simulink model "plant_control"  (R2023a)
settings: Solver=FixedStepAuto  StartTime=0.0  StopTime=10  FixedStep=0.01  RelTol=1e-3
values from neighbouring files (symbols this model uses):
  g = 9.81    [control_params.m]
  Ginv = inv(G)    [control_params.m]
  kF = -9.17e-5    (= -9.17e-05)    [control_params.m]
  kM = 3.24e-6    (= 3.24e-06)    [control_params.m]
  Kp_p = 7.1614    [control_params.m]
  Kp_pitch = 10.84    [control_params.m]
  Kp_q = 7.1614    [control_params.m]
  Kp_r = 3.3884    [control_params.m]
  Kp_roll = 10.84    [control_params.m]
  Kp_vx = -0.3281    [control_params.m]
  Kp_vy = 0.3281    [control_params.m]
  Kp_vz = 100    [control_params.m]
  Kp_x = 1    [control_params.m]
  Kp_y = 1    [control_params.m]
  Kp_yaw = 10.84    [control_params.m]
  Kp_z = 1    [control_params.m]
  lx = 0.4389087297    [control_params.m]
  ly = 0.4389087297    [control_params.m]
  m = 10    [control_params.m]
  Td = 1/3    (= 0.333333333333)    [control_params.m]
  Ti = 5/3    (= 1.66666666667)    [control_params.m]
libraries: slpidlib x3, shared6dof x1, simulink_extras x1, aerolibnav x1, SignalEditorBlockLib x1
settings Model: Creator=timme  LastModifiedBy=timme
settings OptimizationCC: BlockReduction=off  DefaultParameterBehavior=Inlined  BufferReuse=off

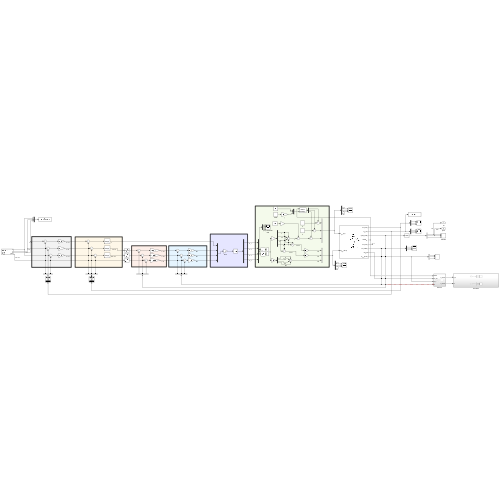
[thumbnail: Simulink's stored preview of the top-level diagram]
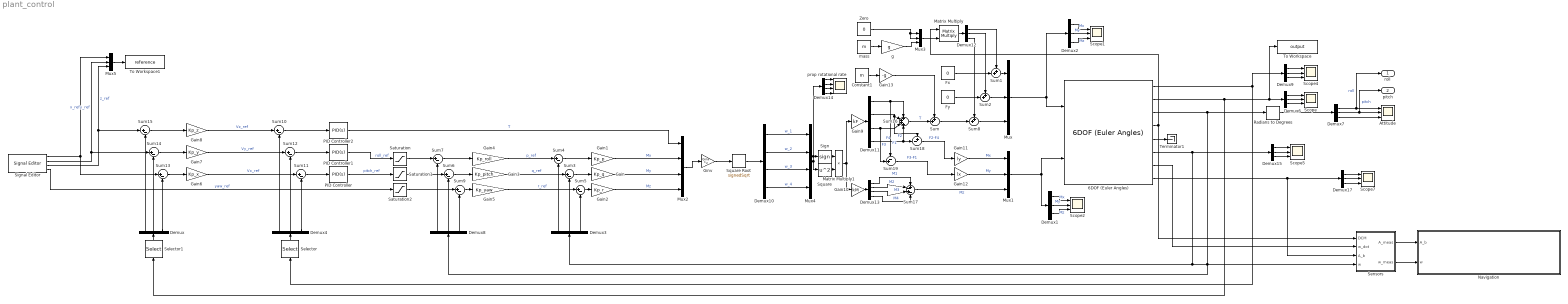
== system plant_control ==
  6DOF (Euler Angles) : shared6dof/6DOF (Euler Angles)  units=Metric (MKS)  mtype=Fixed  rep=Euler Angles  xme_0=[0 0 -1]  Vm_0=[0 0 0]  eul_0=[0 0 0]  pm_0=[0 0 0]  mass_0=m  mass_e=0.5  mass_f=2.0  inertia=I  inertia_e=eye(3)  inertia_f=2*eye(3)  k_quat=1.0  vre_flag=on  abi_flag=off  aMode=0  xme_statename=''  Vm_statename=''  eul_statename=''  quat_statename=''  pm_statename=''  mass_statename=''
  Attitude : Scope  NumInputPorts=3
  Constant1 : Constant  Value=m
  Demux{,1..4,6..9,12,15,17} (12 alike) : Demux  Outputs=3
  Demux{10..11,13..14} (4 alike) : Demux
  Fx : Constant  Value=0
  Fy : Constant  Value=0
  Gain : Gain  Gain=Kp_q
  Gain1 : Gain  Gain=Kp_p
  Gain10 : Gain  Gain=kM
  Gain11 : Gain  Gain=ly
  Gain12 : Gain  Gain=lx
  Gain13 : Gain  Gain=-g
  Gain2 : Gain  Gain=Kp_r
  Gain3 : Gain  Gain=Kp_pitch
  Gain4 : Gain  Gain=Kp_roll
  Gain5 : Gain  Gain=Kp_yaw
  Gain6 : Gain  Gain=Kp_x
  Gain7 : Gain  Gain=Kp_y
  Gain8 : Gain  Gain=Kp_z
  Gain9 : Gain  Gain=kF
  Ginv : Gain  Gain=Ginv  Multiplication=Matrix(K*u)
  Matrix Multiply : Product  Inputs=**  Multiplication=Matrix(*)
  Matrix Multiply1 : Product
  Mux{,1,3,5} (4 alike) : Mux  Inputs=3
  Mux2 : Mux
  Mux4 : Mux
  Navigation : Subsystem
  PID Controller : slpidlib/PID Controller  Controller=PID  Form=Parallel  TimeDomain=Continuous-time  UseExternalTs=off  SampleTime=-1  IntegratorMethod=Forward Euler  FilterMethod=Forward Euler  ControllerParametersSource=internal  P=Kp_vx*(1+Td/Ti)  I=Kp_vx/Ti  UseKiTs=off  D=Kp_vx*Td  N=100  UseFilter=on  TunerSelectOption=Transfer Function Based (PID Tuner App)  InitialConditionSource=internal  InitialConditionForIntegrator=0  InitialConditionForFilter=0  DifferentiatorICPrevScaledInput=0  ExternalReset=none  TrackingMode=off  Kt=1  LimitOutput=off  SatLimitsSource=internal  UpperSaturationLimit=inf  LowerSaturationLimit=-inf  LinearizeAsGain=on  AntiWindupMode=none  Kb=1  LimitIntegrator=off  UpperIntegratorSaturationLimit=inf  LowerIntegratorSaturationLimit=-inf  POutMin=[]  POutMax=[]  IOutMin=[]  IOutMax=[]  DOutMin=[]  DOutMax=[]  NOutMin=[]  NOutMax=[]  SumOutMin=[]  SumOutMax=[]  SaturationOutMin=[]  SaturationOutMax=[]  PParamMin=[]  PParamMax=[]  IParamMin=[]  IParamMax=[]  DParamMin=[]  DParamMax=[]  NParamMin=[]  NParamMax=[]  KbParamMin=[]  KbParamMax=[]  KtParamMin=[]  KtParamMax=[]  KbOutMin=[]  KbOutMax=[]  KtOutMin=[]  KtOutMax=[]  IntegratorOutMin=[]  IntegratorOutMax=[]  FilterOutMin=[]  FilterOutMax=[]  SumI1OutMin=[]  SumI1OutMax=[]  SumI2OutMin=[]  SumI2OutMax=[]  SumI3OutMin=[]  SumI3OutMax=[]  SumI4OutMin=[]  SumI4OutMax=[]  SumDOutMin=[]  SumDOutMax=[]  DifferentiatorOutMin=[]  DifferentiatorOutMax=[]  FilterDiffOutCoefMin=[]  FilterDiffOutCoefMax=[]  ReciprocalOutMin=[]  ReciprocalOutMax=[]  SumDenOutMin=[]  SumDenOutMax=[]  SumNumOutMin=[]  SumNumOutMax=[]  DivideOutMin=[]  DivideOutMax=[]  UdiffTsProdOutMin=[]  UdiffTsProdOutMax=[]  NTsProdOutMin=[]  NTsProdOutMax=[]  UintegralTsProdOutMin=[]  UintegralTsProdOutMax=[]  UngainTsProdOutMin=[]  UngainTsProdOutMax=[]  ClampingZeroOutDataTypeStr=Inherit: Inherit via back propagation  ClampingZeroOutMin=[]  ClampingZeroOutMax=[]  FilterDenConstantOutDataTypeStr=Inherit: Inherit via back propagation  FilterDenConstantOutMin=[]  FilterDenConstantOutMax=[]  PCopyOutDataTypeStr=Inherit: Inherit via back propagation  PCopyOutMin=[]  PCopyOutMax=[]  NCopyOutDataTypeStr=Inherit: Inherit via back propagation  NCopyOutMin=[]  NCopyOutMax=[]  IntegratorContinuousStateAttributes=''  IntegratorStateMustResolveToSignalObject=off  IntegratorRTWStateStorageClass=Auto  FilterContinuousStateAttributes=''  FilterStateMustResolveToSignalObject=off  FilterRTWStateStorageClass=Auto  ParallelPVariant=InternalParameters  IdealPVariant=Disabled  IVariant=InternalParameters  DVariant=InternalParameters  IntegratorVariant=Continuous  SatVariant=Disabled  AWVariant=Passthrough  PCopyVariant=Disabled  TRVariant=Disabled  FdbkBlocksVariant=Forward  IdealPFdbkVariant=Disabled  SatFdbkVariant=Disabled  DerivativeFilterVariant=ContFilter  NVariant=InternalParameters  NCopyVariant=Disabled  FilterICVariant=InternalICsFilter  IntegratorICVariant=InternalICs  ExternalResetVariant=Disabled  TRSumVariant=Passthrough  SumFdbkVariant=Disabled  SumVariant=Sum_PID  TsampFilterVariant=InternalTs  TsampNgainVariant=Passthrough  TsampIntegralVariant=Disabled_SignalSpec  ExternalSaturationOutDataTypeStr=Inherit: Same as second input
  PID Controller1 : slpidlib/PID Controller  Controller=PID  Form=Parallel  TimeDomain=Continuous-time  UseExternalTs=off  SampleTime=-1  IntegratorMethod=Forward Euler  FilterMethod=Forward Euler  ControllerParametersSource=internal  P=Kp_vy*(1+Td/Ti)  I=Kp_vy/Ti  UseKiTs=off  D=Kp_vy*Td  N=100  UseFilter=on  TunerSelectOption=Transfer Function Based (PID Tuner App)  InitialConditionSource=internal  InitialConditionForIntegrator=0  InitialConditionForFilter=0  DifferentiatorICPrevScaledInput=0  ExternalReset=none  TrackingMode=off  Kt=1  LimitOutput=off  SatLimitsSource=internal  UpperSaturationLimit=inf  LowerSaturationLimit=-inf  LinearizeAsGain=on  AntiWindupMode=none  Kb=1  LimitIntegrator=off  UpperIntegratorSaturationLimit=inf  LowerIntegratorSaturationLimit=-inf  POutMin=[]  POutMax=[]  IOutMin=[]  IOutMax=[]  DOutMin=[]  DOutMax=[]  NOutMin=[]  NOutMax=[]  SumOutMin=[]  SumOutMax=[]  SaturationOutMin=[]  SaturationOutMax=[]  PParamMin=[]  PParamMax=[]  IParamMin=[]  IParamMax=[]  DParamMin=[]  DParamMax=[]  NParamMin=[]  NParamMax=[]  KbParamMin=[]  KbParamMax=[]  KtParamMin=[]  KtParamMax=[]  KbOutMin=[]  KbOutMax=[]  KtOutMin=[]  KtOutMax=[]  IntegratorOutMin=[]  IntegratorOutMax=[]  FilterOutMin=[]  FilterOutMax=[]  SumI1OutMin=[]  SumI1OutMax=[]  SumI2OutMin=[]  SumI2OutMax=[]  SumI3OutMin=[]  SumI3OutMax=[]  SumI4OutMin=[]  SumI4OutMax=[]  SumDOutMin=[]  SumDOutMax=[]  DifferentiatorOutMin=[]  DifferentiatorOutMax=[]  FilterDiffOutCoefMin=[]  FilterDiffOutCoefMax=[]  ReciprocalOutMin=[]  ReciprocalOutMax=[]  SumDenOutMin=[]  SumDenOutMax=[]  SumNumOutMin=[]  SumNumOutMax=[]  DivideOutMin=[]  DivideOutMax=[]  UdiffTsProdOutMin=[]  UdiffTsProdOutMax=[]  NTsProdOutMin=[]  NTsProdOutMax=[]  UintegralTsProdOutMin=[]  UintegralTsProdOutMax=[]  UngainTsProdOutMin=[]  UngainTsProdOutMax=[]  ClampingZeroOutDataTypeStr=Inherit: Inherit via back propagation  ClampingZeroOutMin=[]  ClampingZeroOutMax=[]  FilterDenConstantOutDataTypeStr=Inherit: Inherit via back propagation  FilterDenConstantOutMin=[]  FilterDenConstantOutMax=[]  PCopyOutDataTypeStr=Inherit: Inherit via back propagation  PCopyOutMin=[]  PCopyOutMax=[]  NCopyOutDataTypeStr=Inherit: Inherit via back propagation  NCopyOutMin=[]  NCopyOutMax=[]  IntegratorContinuousStateAttributes=''  IntegratorStateMustResolveToSignalObject=off  IntegratorRTWStateStorageClass=Auto  FilterContinuousStateAttributes=''  FilterStateMustResolveToSignalObject=off  FilterRTWStateStorageClass=Auto  ParallelPVariant=InternalParameters  IdealPVariant=Disabled  IVariant=InternalParameters  DVariant=InternalParameters  IntegratorVariant=Continuous  SatVariant=Disabled  AWVariant=Passthrough  PCopyVariant=Disabled  TRVariant=Disabled  FdbkBlocksVariant=Forward  IdealPFdbkVariant=Disabled  SatFdbkVariant=Disabled  DerivativeFilterVariant=ContFilter  NVariant=InternalParameters  NCopyVariant=Disabled  FilterICVariant=InternalICsFilter  IntegratorICVariant=InternalICs  ExternalResetVariant=Disabled  TRSumVariant=Passthrough  SumFdbkVariant=Disabled  SumVariant=Sum_PID  TsampFilterVariant=InternalTs  TsampNgainVariant=Passthrough  TsampIntegralVariant=Disabled_SignalSpec  ExternalSaturationOutDataTypeStr=Inherit: Same as second input
  PID Controller2 : slpidlib/PID Controller  Controller=PID  Form=Parallel  TimeDomain=Continuous-time  UseExternalTs=off  SampleTime=-1  IntegratorMethod=Forward Euler  FilterMethod=Forward Euler  ControllerParametersSource=internal  P=Kp_vz  I=50  UseKiTs=off  D=0  N=100  UseFilter=on  TunerSelectOption=Transfer Function Based (PID Tuner App)  InitialConditionSource=internal  InitialConditionForIntegrator=0  InitialConditionForFilter=0  DifferentiatorICPrevScaledInput=0  ExternalReset=none  TrackingMode=off  Kt=1  LimitOutput=off  SatLimitsSource=internal  UpperSaturationLimit=inf  LowerSaturationLimit=-inf  LinearizeAsGain=on  AntiWindupMode=none  Kb=1  LimitIntegrator=off  UpperIntegratorSaturationLimit=inf  LowerIntegratorSaturationLimit=-inf  POutMin=[]  POutMax=[]  IOutMin=[]  IOutMax=[]  DOutMin=[]  DOutMax=[]  NOutMin=[]  NOutMax=[]  SumOutMin=[]  SumOutMax=[]  SaturationOutMin=[]  SaturationOutMax=[]  PParamMin=[]  PParamMax=[]  IParamMin=[]  IParamMax=[]  DParamMin=[]  DParamMax=[]  NParamMin=[]  NParamMax=[]  KbParamMin=[]  KbParamMax=[]  KtParamMin=[]  KtParamMax=[]  KbOutMin=[]  KbOutMax=[]  KtOutMin=[]  KtOutMax=[]  IntegratorOutMin=[]  IntegratorOutMax=[]  FilterOutMin=[]  FilterOutMax=[]  SumI1OutMin=[]  SumI1OutMax=[]  SumI2OutMin=[]  SumI2OutMax=[]  SumI3OutMin=[]  SumI3OutMax=[]  SumI4OutMin=[]  SumI4OutMax=[]  SumDOutMin=[]  SumDOutMax=[]  DifferentiatorOutMin=[]  DifferentiatorOutMax=[]  FilterDiffOutCoefMin=[]  FilterDiffOutCoefMax=[]  ReciprocalOutMin=[]  ReciprocalOutMax=[]  SumDenOutMin=[]  SumDenOutMax=[]  SumNumOutMin=[]  SumNumOutMax=[]  DivideOutMin=[]  DivideOutMax=[]  UdiffTsProdOutMin=[]  UdiffTsProdOutMax=[]  NTsProdOutMin=[]  NTsProdOutMax=[]  UintegralTsProdOutMin=[]  UintegralTsProdOutMax=[]  UngainTsProdOutMin=[]  UngainTsProdOutMax=[]  ClampingZeroOutDataTypeStr=Inherit: Inherit via back propagation  ClampingZeroOutMin=[]  ClampingZeroOutMax=[]  FilterDenConstantOutDataTypeStr=Inherit: Inherit via back propagation  FilterDenConstantOutMin=[]  FilterDenConstantOutMax=[]  PCopyOutDataTypeStr=Inherit: Inherit via back propagation  PCopyOutMin=[]  PCopyOutMax=[]  NCopyOutDataTypeStr=Inherit: Inherit via back propagation  NCopyOutMin=[]  NCopyOutMax=[]  IntegratorContinuousStateAttributes=''  IntegratorStateMustResolveToSignalObject=off  IntegratorRTWStateStorageClass=Auto  FilterContinuousStateAttributes=''  FilterStateMustResolveToSignalObject=off  FilterRTWStateStorageClass=Auto  ParallelPVariant=InternalParameters  IdealPVariant=Disabled  IVariant=InternalParameters  DVariant=InternalParameters  IntegratorVariant=Continuous  SatVariant=Disabled  AWVariant=Passthrough  PCopyVariant=Disabled  TRVariant=Disabled  FdbkBlocksVariant=Forward  IdealPFdbkVariant=Disabled  SatFdbkVariant=Disabled  DerivativeFilterVariant=ContFilter  NVariant=InternalParameters  NCopyVariant=Disabled  FilterICVariant=InternalICsFilter  IntegratorICVariant=InternalICs  ExternalResetVariant=Disabled  TRSumVariant=Passthrough  SumFdbkVariant=Disabled  SumVariant=Sum_PID  TsampFilterVariant=InternalTs  TsampNgainVariant=Passthrough  TsampIntegralVariant=Disabled_SignalSpec  ExternalSaturationOutDataTypeStr=Inherit: Same as second input
  Radians to Degrees : simulink_extras/Transformations/Radians to Degrees
  Saturation : Saturate  UpperLimit=pi/3  LowerLimit=-pi/3
  Saturation1 : Saturate  UpperLimit=pi/3  LowerLimit=-pi/3
  Saturation2 : Saturate  UpperLimit=pi  LowerLimit=-pi
  Scope{,1..2,4..5,7} (6 alike) : Scope  NumInputPorts=3
  Selector : Selector  InputPortWidth=3  IndexOptions=Index vector (dialog)  Indices=[3 2 1]  OutputSizes=1
  Selector1 : Selector  InputPortWidth=3  IndexOptions=Index vector (dialog)  Indices=[3 2 1]  OutputSizes=1
  Sensors : Subsystem
  Sign : Signum
  Signal Editor : SignalEditorBlockLib/Signal Editor  FileName=C:\Users\timme\OneDrive\Bureaublad\Tu Delft\bsc3\DSE\GNC development\Conceptual design phase\Test files\full_system_reference.mat  ActiveScenario=flightZ_dir  ActiveSignal=z  IsBus=off  OutputBusObjectStr=Bus: BusObject  SampleTime=0  Interpolate=off  ZeroCross=off  OutputAfterFinalValue=Setting to zero  Unit=inherit  PreserveSignalName=on  ApplySigPropsToAllScenarios=on
  Square : Math  Operator=square
  Square Root : Sqrt  Operator=signedSqrt  OutputSignalType=real
  Sum{,1..2,8} (4 alike) : Sum  Inputs=++|
  Sum{3..7,9..15} (12 alike) : Sum  Inputs=|+-
  Sum16 : Sum  Inputs=++++
  Sum17 : Sum  Inputs=+-+-
  Sum18 : Sum  Inputs=+-|
  Sum19 : Sum  Inputs=-+|
  Terminator1 : Terminator
  To Workspace : ToWorkspace  VariableName=output  SaveFormat=Timeseries  SampleTime=-1
  To Workspace1 : ToWorkspace  VariableName=reference  SaveFormat=Timeseries  SampleTime=-1
  Zero : Constant  Value=0  OutDataTypeStr=Inherit: Inherit via back propagation
  g : Gain  Gain=g
  mass : Constant  Value=m
  prop rotational rate : Scope  NumInputPorts=4
  roll : Outport
  pitch : Outport  Port=2
  wires:
  Mux1/1 -> 6DOF (Euler Angles)/2, Demux1/1
  6DOF (Euler Angles)/5 -> Terminator1/1
  Demux1/2 -> Scope2/2  "My"
  Demux1/1 -> Scope2/1  "Mx"
  Demux1/3 -> Scope2/3  "Mz"
  Gain/1 -> Mux2/3  "My"
  mass/1 -> g/1
  Zero/1 -> Mux3/1, Mux3/2
  Sum2/1 -> Mux/2
  6DOF (Euler Angles)/4 -> Sensors/1(DCM), Matrix Multiply/1
  Fx/1 -> Sum1/2
  Demux12/1 -> Sum1/1
  g/1 -> Mux3/3
  Sum8/1 -> Mux/3
  Matrix Multiply/1 -> Demux12/1
  Sum16/1 -> Sum/2  "T"
  Sum1/1 -> Mux/1
  Demux12/3 -> Sum8/1
  Fy/1 -> Sum2/2
  Mux3/1 -> Matrix Multiply/2
  Demux12/2 -> Sum2/1
  Mux/1 -> Demux2/1, 6DOF (Euler Angles)/1
  Demux2/1 -> Scope1/1  "Mx"
  Demux2/2 -> Scope1/2  "My"
  Demux2/3 -> Scope1/3  "Mz"
  Sum3/1 -> Gain/1
  Sum4/1 -> Gain1/1
  Sum5/1 -> Gain2/1
  6DOF (Euler Angles)/6 -> Demux3/1, Sensors/4(w), Demux15/1
  Sum6/1 -> Gain3/1
  Sum7/1 -> Gain4/1
  Gain5/1 -> Sum5/1  "r_ref"
  Gain4/1 -> Sum4/1  "p_ref"
  Gain3/1 -> Sum3/1  "q_ref"
  Sum9/1 -> Gain5/1
  PID Controller1/1 -> Saturation/1  "roll_ref"
  Gain8/1 -> Sum10/1  "Vz_ref"
  Demux4/2 -> Sum12/2
  6DOF (Euler Angles)/1 -> Selector/1, Demux9/1
  Demux4/3 -> Sum11/2
  Sum11/1 -> PID Controller/1
  Sum13/1 -> Gain6/1
  PID Controller/1 -> Saturation1/1  "pitch_ref"
  Selector/1 -> Demux4/1
  Demux4/1 -> Sum10/2
  Gain7/1 -> Sum12/1  "Vy_ref"
  Sum12/1 -> PID Controller1/1
  PID Controller2/1 -> Mux2/1  "T"
  Signal Editor/4 -> Saturation2/1  "yaw_ref"
  Sum10/1 -> PID Controller2/1
  Demux8/3 -> Sum9/2
  Demux8/2 -> Sum6/2
  Demux8/1 -> Sum7/2
  Demux3/3 -> Sum5/2
  Demux3/2 -> Sum3/2
  Demux3/1 -> Sum4/2
  Demux/3 -> Sum13/2
  Gain6/1 -> Sum11/1  "Vx_ref"
  Selector1/1 -> Demux/1
  Demux/2 -> Sum14/2
  Sum14/1 -> Gain7/1
  Demux/1 -> Sum15/2
  Sum15/1 -> Gain8/1
  Signal Editor/2 -> Mux5/2, Sum14/1  "y_ref"
  Signal Editor/3 -> Mux5/3, Sum15/1  "z_ref"
  Signal Editor/1 -> Sum13/1, Mux5/1  "x_ref"
  Demux6/2 -> Scope/2
  Demux6/1 -> Scope/1
  Demux6/3 -> Scope/3
  Demux7/2 -> pitch/1, Attitude/2  "pitch"
  Demux7/3 -> Attitude/3
  Demux7/1 -> roll/1, Attitude/1  "roll"
  Radians to Degrees/1 -> Demux7/1
  Demux9/2 -> Scope4/2
  Demux9/3 -> Scope4/3
  Demux9/1 -> Scope4/1
  Gain1/1 -> Mux2/2  "Mx"
  Gain2/1 -> Mux2/4  "Mz"
  Mux2/1 -> Ginv/1
  Ginv/1 -> Square Root/1
  Demux10/1 -> Mux4/1  "w_1"
  Demux10/2 -> Mux4/2  "w_2"
  Demux10/3 -> Mux4/3  "w_3"
  Demux10/4 -> Mux4/4  "w_4"
  Gain9/1 -> Demux11/1
  Demux11/1 -> Sum19/1, Sum16/1  "F1"
  Demux11/2 -> Sum18/1, Sum16/2  "F2"
  Demux11/3 -> Sum19/2, Sum16/3  "F3"
  Demux11/4 -> Sum18/2, Sum16/4  "F4"
  Demux13/4 -> Sum17/4  "M4"
  Demux13/3 -> Sum17/3  "M3"
  Demux13/2 -> Sum17/2  "M2"
  Gain10/1 -> Demux13/1
  Demux13/1 -> Sum17/1  "M1"
  Sum17/1 -> Mux1/3  "Mz"
  Sum18/1 -> Gain11/1  "F2-F4"
  Gain11/1 -> Mux1/1  "Mx"
  Sum19/1 -> Gain12/1  "F3-F1"
  Gain12/1 -> Mux1/2  "My"
  Square Root/1 -> Demux10/1
  Mux4/1 -> Demux14/1, Sign/1, Square/1
  Sign/1 -> Matrix Multiply1/1
  Square/1 -> Matrix Multiply1/2
  Matrix Multiply1/1 -> Gain9/1, Gain10/1
  Demux14/2 -> prop rotational rate/2
  Demux14/1 -> prop rotational rate/1
  Demux14/3 -> prop rotational rate/3
  Demux14/4 -> prop rotational rate/4
  6DOF (Euler Angles)/2 -> Selector1/1, To Workspace/1, Demux6/1
  6DOF (Euler Angles)/3 -> Radians to Degrees/1, Demux8/1
  Saturation/1 -> Sum7/1
  Saturation1/1 -> Sum6/1
  Saturation2/1 -> Sum9/1
  Constant1/1 -> Gain13/1
  Gain13/1 -> Sum/1
  Sum/1 -> Sum8/2
  Mux5/1 -> To Workspace1/1
  6DOF (Euler Angles)/7 -> Sensors/2(w_dot)
  6DOF (Euler Angles)/8 -> Sensors/3(A_b), Demux17/1
  Demux15/2 -> Scope5/2
  Demux15/3 -> Scope5/3
  Demux15/1 -> Scope5/1
  Demux17/1 -> Scope7/1
  Demux17/2 -> Scope7/2
  Demux17/3 -> Scope7/3
  Sensors/1(A_meas) -> Navigation/1(A_b)
  Sensors/2(w_meas) -> Navigation/2(w)

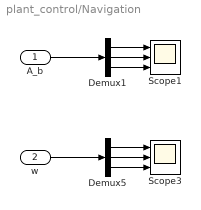
== system plant_control/Navigation ==
  A_b : Inport
  w : Inport  Port=2
  Demux1 : Demux  Outputs=3
  Demux5 : Demux  Outputs=3
  Scope1 : Scope  NumInputPorts=3
  Scope3 : Scope  NumInputPorts=3
  wires:
  Demux5/1 -> Scope3/1
  Demux5/3 -> Scope3/3
  Demux5/2 -> Scope3/2
  Demux1/3 -> Scope1/3
  Demux1/1 -> Scope1/1
  Demux1/2 -> Scope1/2
  A_b/1 -> Demux1/1
  w/1 -> Demux5/1

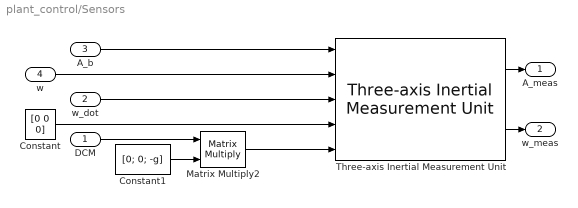
== system plant_control/Sensors ==
  DCM : Inport
  w_dot : Inport  Port=2
  A_b : Inport  Port=3
  w : Inport  Port=4
  Constant : Constant  Value=[0 0 0]
  Constant1 : Constant  Value=[0; 0; -g]
  Matrix Multiply2 : Product  Inputs=**  Multiplication=Matrix(*)
  Three-axis Inertial Measurement Unit : aerolibnav/Three-axis Inertial Measurement Unit  units=Metric (MKS)  imu=[0 0 0]  i_Ts=0.01  dtype_a=on  w_a=190  z_a=0.707  a_sf_cc=[1 0 0; 0 1 0; 0 0 1]  a_bias=[0 0 0]  a_sat="[-inf  -inf  -inf  inf inf inf]"  dtype_g=on  w_g=190  z_g=0.707  g_sf_cc=[1 0 0; 0 1 0; 0 0 1]  g_bias=[0 0 0]  g_sens=[0 0 0]  g_sat="[-inf  -inf  -inf  inf inf inf]"  i_rand=on  i_seeds=[23093 23094 23095 23096 23097 23098]  i_pow=[0.001 0.001 0.001 0.0001 0.0001 0.0001]
  A_meas : Outport
  w_meas : Outport  Port=2
  wires:
  Constant1/1 -> Matrix Multiply2/2
  Constant/1 -> Three-axis Inertial Measurement Unit/4
  Three-axis Inertial Measurement Unit/1 -> A_meas/1
  DCM/1 -> Matrix Multiply2/1
  Three-axis Inertial Measurement Unit/2 -> w_meas/1
  A_b/1 -> Three-axis Inertial Measurement Unit/1
  w/1 -> Three-axis Inertial Measurement Unit/2
  w_dot/1 -> Three-axis Inertial Measurement Unit/3
  Matrix Multiply2/1 -> Three-axis Inertial Measurement Unit/5
